simulink model "Model"  (R2014b)
settings: Solver=ode45  StartTime=0.0  StopTime=10.0  RelTol=1e-3
values from neighbouring files (symbols this model uses):
  dt = 9.2e6    (= 9200000)    [Parameters.m]
  Jpp = 1e6    (= 1000000)    [Parameters.m]
  Jt = 1.56e8    (= 156000000)    [Parameters.m]
  kt = 2.3e9    (= 2300000000)    [Parameters.m]
  phs = 40    [Parameters.m]
  Q = G    (= 7.5)    [Parameters.m]
  Tpull = 11.9e6    (= 11900000)    [Parameters.m]
settings Model: Creator=Eduardo Montilva  LastModifiedBy=Eduardo Montilva

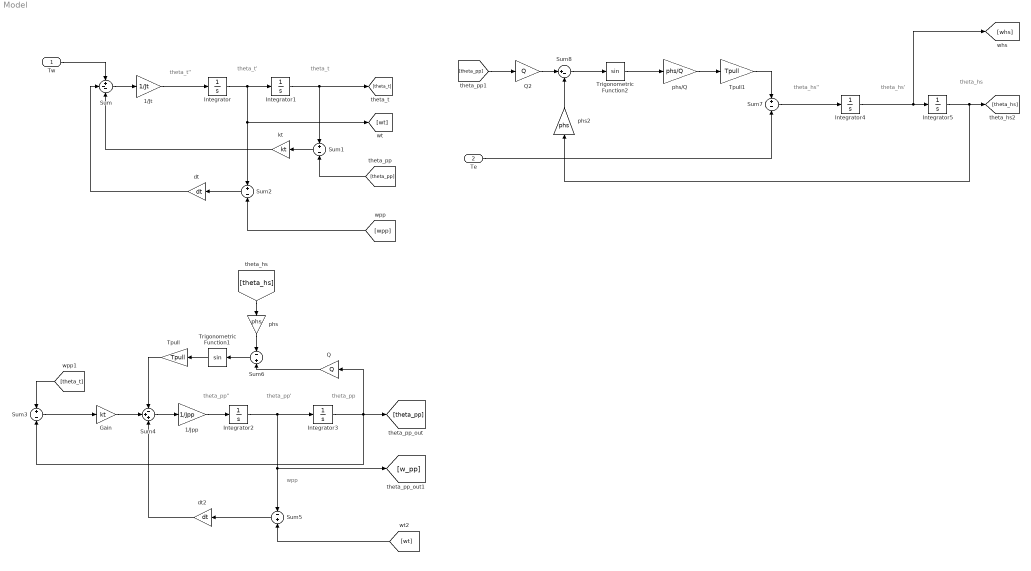
== system Model ==
  note: theta_hs
  note: theta_hs'
  note: theta_hs''
  note: theta_pp
  note: wpp
  note: theta_pp'
  note: theta_pp''
  note: theta_t
  note: theta_t'
  note: theta_t''
  Tw : Inport
  Te : Inport  Port=2
  1/Jpp : Gain  Gain=1/Jpp
  1/Jt : Gain  Gain=1/Jt
  Gain : Gain  Gain=kt
  Integrator{,1..5} (6 alike) : Integrator
  Q : Gain  Gain=Q
  Q2 : Gain  Gain=Q
  Sum : Sum  Inputs=+--
  Sum1 : Sum  Inputs=+-
  Sum2 : Sum  Inputs=+-
  Sum3 : Sum  Inputs=+|-
  Sum4 : Sum  Inputs=-++
  Sum5 : Sum  Inputs=-+
  Sum6 : Sum  Inputs=-|+
  Sum7 : Sum  Inputs=+-
  Sum8 : Sum  Inputs=|+-
  Tpull : Gain  Gain=Tpull
  Tpull1 : Gain  Gain=Tpull
  Trigonometric Function1 : Trigonometry
  Trigonometric Function2 : Trigonometry
  dt : Gain  Gain=dt
  dt2 : Gain  Gain=dt
  kt : Gain  Gain=kt
  phs : Gain  Gain=phs
  phs/Q : Gain  Gain=phs/Q
  phs2 : Gain  Gain=phs
  wires:
  Sum/1 -> 1/Jt/1
  1/Jt/1 -> Integrator/1
  Integrator1/1 -> [theta_t], Sum1/1
  [theta_pp] -> Sum1/2
  Sum1/1 -> kt/1
  Tw/1 -> Sum/1
  kt/1 -> Sum/3
  Integrator/1 -> Sum2/1, [wt], Integrator1/1
  [wpp] -> Sum2/2
  Sum2/1 -> dt/1
  dt/1 -> Sum/2
  [theta_t] -> Sum3/1
  Sum3/1 -> Gain/1
  Gain/1 -> Sum4/2
  Sum4/1 -> 1/Jpp/1
  1/Jpp/1 -> Integrator2/1
  Integrator3/1 -> Sum3/2, Q/1, [theta_pp]
  Integrator2/1 -> [w_pp], Sum5/1, Integrator3/1
  Sum5/1 -> dt2/1
  dt2/1 -> Sum4/3
  Q/1 -> Sum6/2
  [theta_hs] -> phs/1
  phs/1 -> Sum6/1
  Sum6/1 -> Trigonometric Function1/1
  Trigonometric Function1/1 -> Tpull/1
  Tpull/1 -> Sum4/1
  [wt] -> Sum5/2
  phs/Q/1 -> Tpull1/1
  Tpull1/1 -> Sum7/1
  Te/1 -> Sum7/2
  Q2/1 -> Sum8/1
  [theta_pp] -> Q2/1
  phs2/1 -> Sum8/2
  Sum8/1 -> Trigonometric Function2/1
  Trigonometric Function2/1 -> phs/Q/1
  Sum7/1 -> Integrator4/1
  Integrator4/1 -> [whs], Integrator5/1
  Integrator5/1 -> phs2/1, [theta_hs]
